simulink model "test"  (R2021a)
settings: Solver=VariableStepAuto  StartTime=0.0  StopTime=10.0  RelTol=1e-3
settings Model: Creator=pierr  LastModifiedBy=pierr

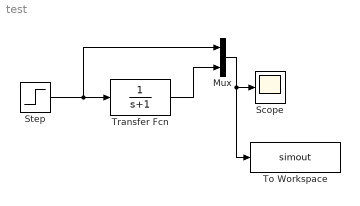
== system test ==
  Mux : Mux  Inputs=2
  Scope : Scope
  Step : Step  SampleTime=0
  To Workspace : ToWorkspace  VariableName=simout  SampleTime=-1
  Transfer Fcn : TransferFcn  Denominator=[1 1]
  wires:
  Transfer Fcn/1 -> Mux/2
  Mux/1 -> To Workspace/1, Scope/1
  Step/1 -> Mux/1, Transfer Fcn/1
